simulink model "arm_sim"  (R2018b)
settings: Solver=ode45  StartTime=0.0  StopTime=10000  RelTol=1e-3  EnableMultiTasking=on
InitFcn:
  | addpath ./..
  | arm_param
undefined symbols (not defined in the file): P
libraries: simulink x1
settings Model: Creator=beard  LastModifiedBy=beard
settings DataIOCC: LimitDataPoints=on  SaveFormat=Array  SignalLoggingSaveFormat=ModelDataLogs
settings OptimizationCC: ExpressionDepthLimit=2147483647  InitFltsAndDblsToZero=on  LifeSpan=inf
settings DebuggingCC: UnderspecifiedInitializationDetection=Classic  MergeDetectMultiDrivingBlocksExec=none  SolverPrmCheckMsg=warning  FcnCallInpInsideContextMsg=warning  StateNameClashWarn=warning  SFUnexpectedBacktrackingDiag=warning  SFNoUnconditionalDefaultTransitionDiag=warning  SFExecutionAtInitializationDiag=none
settings HardwareCC: ProdBitPerPointer=32  ProdBitPerSizeT=32  ProdBitPerPtrDiffT=32  ProdLargestAtomicFloat=None  ProdIntDivRoundTo=Undefined  ProdEndianess=Unspecified  ProdWordSize=32  ProdHWDeviceType=32-bit Generic
settings ModelReferenceCC: PropagateSignalLabelsOutOfModel=off
settings SFSimCC: SimUseLocalCustomCode=off
settings RTWCC: RTWUseLocalCustomCode=off
settings CodeAppCC: StateflowObjectComments=on
settings GRTTargetCC: TargetLangStandard=C89/C90 (ANSI)  GeneratePreprocessorConditionals=Disable all  CombineOutputUpdateFcns=off  GRTInterface=on
settings ConfigComp: CovMetricSettings=dw  CovHtmlReporting=on  CovSaveCumulativeToWorkspaceVar=on  CovSaveSingleToWorkspaceVar=on  CovExternalEMLEnable=off

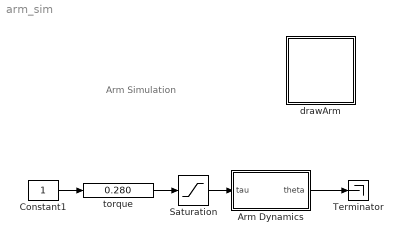
== system arm_sim ==
  note: Arm Simulation
  "Arm Dynamics " : Subsystem
  Constant1 : Constant
  Saturation : Saturate  UpperLimit=P.tau_max  LowerLimit=-P.tau_max
  Terminator : Terminator
  drawArm : Subsystem
      mask Display: image(imread('tv.jpg'))
  torque : simulink/Math Operations/Slider Gain  gain=0.280  low=-1  high=1
  wires:
  Constant1/1 -> torque/1
  "Arm Dynamics "/1("theta ") -> Terminator/1
  torque/1 -> Saturation/1
  Saturation/1 -> "Arm Dynamics "/1(tau)

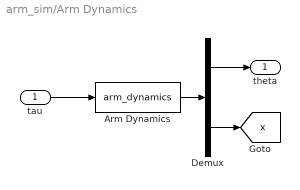
== system arm_sim/Arm Dynamics  ==
  tau : Inport
  Arm Dynamics : S-Function  FunctionName=arm_dynamics  Parameters=P  SFunctionDeploymentMode=off  EnableBusSupport=off
  Demux : Demux  Outputs=[1;2]
  "theta " : Outport
  tag scope: x=global
  wires:
  tau/1 -> Arm Dynamics/1
  Demux/1 -> "theta "/1
  Demux/2 -> [x]
  Arm Dynamics/1 -> Demux/1

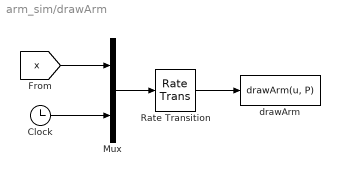
== system arm_sim/drawArm ==
  Clock : Clock
  Mux : Mux  Inputs=2
  Rate Transition : RateTransition  OutPortSampleTime=P.t_plot
  drawArm : MATLABFcn  MATLABFcn=drawArm(u, P)  OutputDimensions=0
  wires:
  Rate Transition/1 -> drawArm/1
  Mux/1 -> Rate Transition/1
  Clock/1 -> Mux/2
  [x] -> Mux/1
